simulink model "HW2_2"  (R2021a)
settings: Solver=VariableStepAuto  StartTime=0.0  StopTime=2  RelTol=1e-3
settings Model: Creator=jhart  LastModifiedBy=jhart

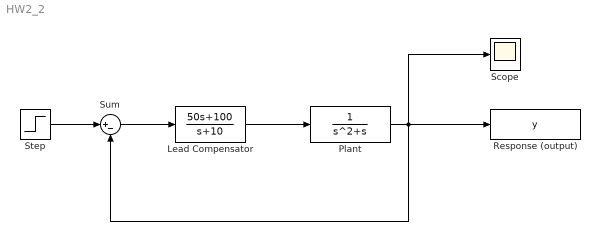
== system HW2_2 ==
  Lead Compensator : TransferFcn  Numerator=[50 100]  Denominator=[1 10]
  Plant : TransferFcn  Denominator=[1 1 0]
  Response (output) : ToWorkspace  VariableName=y  SaveFormat=Timeseries  SampleTime=-1
  Scope : Scope
  Step : Step  Time=0  SampleTime=0
  Sum : Sum  Inputs=|+-
  wires:
  Step/1 -> Sum/1
  Sum/1 -> Lead Compensator/1
  Lead Compensator/1 -> Plant/1
  Plant/1 -> Scope/1, Sum/2, Response (output)/1
